simulink model "P_2_1_l_Kosarlabda_elkapasa"  (R2021b)
settings: Solver=ode5  StartTime=0.0  StopTime=1  FixedStep=0.01  RelTol=1e-3
model workspace (MAT data in the model file):
  tf = Simulink.Parameter
  tf.DataType = 'auto'
  tf.Complexity = 'real'
  tf.Dimensions = [0 0]
undefined symbols (not defined in the file): A_ball, ball_mass, cart_mass, Cd, F0, g, ro_air, theta_0, v0, x_dot_max
settings Model: Creator=davidpaksi  LastModifiedBy=davidpaksi

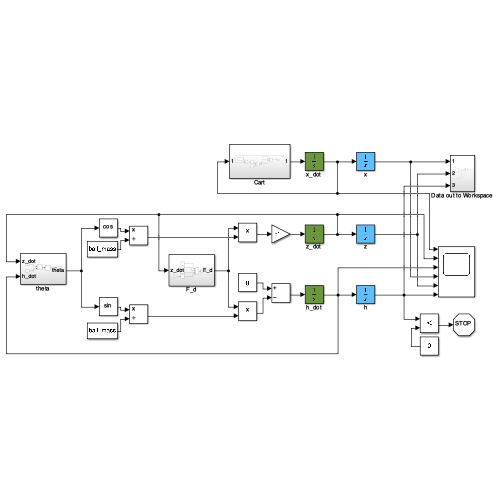
[thumbnail: Simulink's stored preview of the top-level diagram]
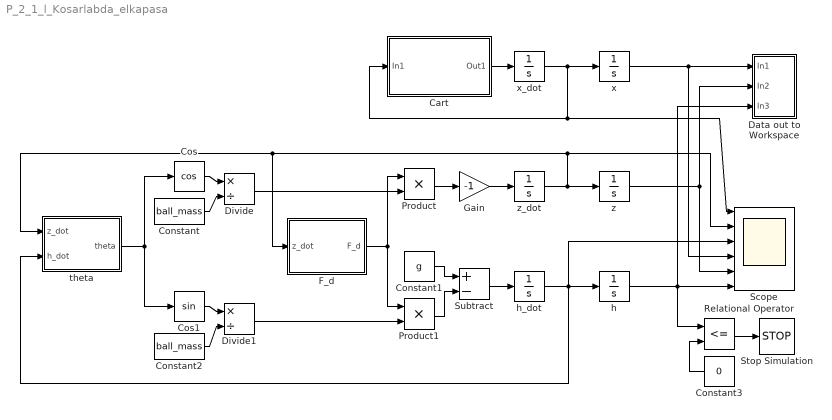
== system P_2_1_l_Kosarlabda_elkapasa ==
  Cart : Subsystem
  Constant : Constant  Value=ball_mass
  Constant1 : Constant  Value=g
  Constant2 : Constant  Value=ball_mass
  Constant3 : Constant  Value=0
  Cos : Trigonometry  Operator=cos
  Cos1 : Trigonometry
  Data out to Workspace : Subsystem
  Divide : Product  Inputs=*/
  Divide1 : Product  Inputs=*/
  F_d : Subsystem
  Gain : Gain  Gain=-1
  Product : Product
  Product1 : Product
  Relational Operator : RelationalOperator  Operator=<=  OutDataTypeStr=boolean  RndMeth=Simplest
  Scope : Scope  NumInputPorts=6
  Stop Simulation : Stop
  Subtract : Sum  Inputs=+-
  h : Integrator  InitialCondition=0.3
  h_dot : Integrator  InitialCondition=sin(theta_0)/cos(theta_0)*v0
  theta : Subsystem
  x : Integrator
  x_dot : Integrator
  z : Integrator  InitialCondition=0.3
  z_dot : Integrator  InitialCondition=v0
  wires:
  z_dot/1 -> Scope/2, theta/1(z_dot), F_d/1(z_dot), z/1
  h_dot/1 -> Scope/3, theta/2(h_dot), h/1
  Gain/1 -> z_dot/1
  Product/1 -> Gain/1
  Constant/1 -> Divide/2
  Cos/1 -> Divide/1
  theta/1(theta) -> Cos1/1, Cos/1
  Divide/1 -> Product/2
  F_d/1(F_d) -> Product1/1, Product/1
  Subtract/1 -> h_dot/1
  Constant1/1 -> Subtract/1
  Constant2/1 -> Divide1/2
  Divide1/1 -> Product1/2
  Cos1/1 -> Divide1/1
  Product1/1 -> Subtract/2
  h/1 -> Relational Operator/1, Data out to Workspace/3(In3), Scope/6
  Constant3/1 -> Relational Operator/2
  Relational Operator/1 -> Stop Simulation/1
  x_dot/1 -> Cart/1(In1), Scope/1, x/1
  x/1 -> Scope/4, Data out to Workspace/1(In1)
  z/1 -> Data out to Workspace/2(In2), Scope/5
  Cart/1(Out1) -> x_dot/1

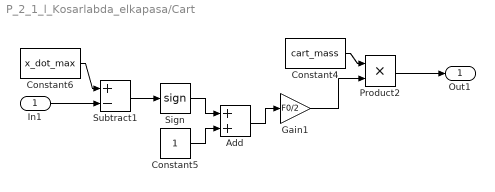
== system P_2_1_l_Kosarlabda_elkapasa/Cart ==
  In1 : Inport
  Add : Sum
  Constant4 : Constant  Value=cart_mass
  Constant5 : Constant
  Constant6 : Constant  Value=x_dot_max
  Gain1 : Gain  Gain=F0/2
  Product2 : Product
  Sign : Signum
  Subtract1 : Sum  Inputs=+-
  Out1 : Outport
  wires:
  Sign/1 -> Add/1
  In1/1 -> Subtract1/2
  Add/1 -> Gain1/1
  Product2/1 -> Out1/1
  Subtract1/1 -> Sign/1
  Constant5/1 -> Add/2
  Constant4/1 -> Product2/1
  Gain1/1 -> Product2/2
  Constant6/1 -> Subtract1/1

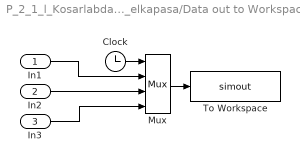
== system P_2_1_l_Kosarlabda_elkapasa/Data out to Workspace ==
  In1 : Inport
  In2 : Inport  Port=2
  In3 : Inport  Port=3
  Clock : Clock
  Mux : Mux
  To Workspace : ToWorkspace  VariableName=simout  SaveFormat=Timeseries  SampleTime=-1
  wires:
  In2/1 -> Mux/3
  In1/1 -> Mux/2
  In3/1 -> Mux/4
  Clock/1 -> Mux/1
  Mux/1 -> To Workspace/1

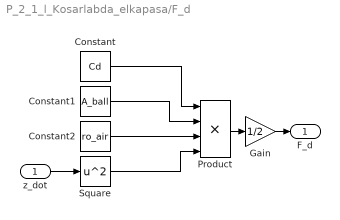
== system P_2_1_l_Kosarlabda_elkapasa/F_d ==
  z_dot : Inport
  Constant : Constant  Value=Cd
  Constant1 : Constant  Value=A_ball
  Constant2 : Constant  Value=ro_air
  Gain : Gain  Gain=1/2
  Product : Product  Inputs=4
  Square : Math  Operator=square  SaturateOnIntegerOverflow=on
  F_d : Outport
  wires:
  Product/1 -> Gain/1
  Gain/1 -> F_d/1
  Constant/1 -> Product/1
  Constant1/1 -> Product/2
  Constant2/1 -> Product/3
  z_dot/1 -> Square/1
  Square/1 -> Product/4

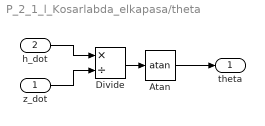
== system P_2_1_l_Kosarlabda_elkapasa/theta ==
  z_dot : Inport
  h_dot : Inport  Port=2
  Atan : Trigonometry  Operator=atan
  Divide : Product  Inputs=*/
  theta : Outport
  wires:
  h_dot/1 -> Divide/1
  Atan/1 -> theta/1
  z_dot/1 -> Divide/2
  Divide/1 -> Atan/1
